simulink model "Uni2Diff"  (R2021b)
settings: Solver=VariableStepAuto  StartTime=0.0  StopTime=10.0  RelTol=1e-3
settings Model: Creator=ericp  LastModifiedBy=ericp

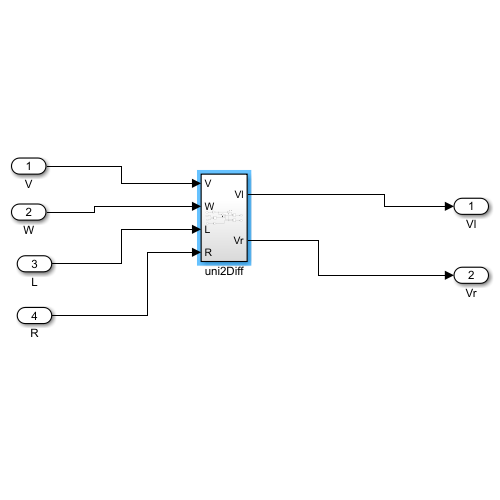
[thumbnail: Simulink's stored preview of the top-level diagram]
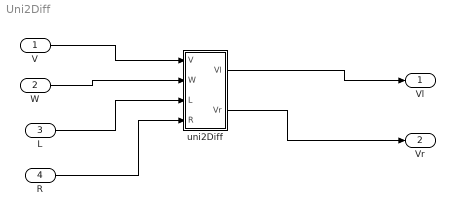
== system Uni2Diff ==
  V : Inport
  W : Inport  Port=2
  L : Inport  Port=3
  R : Inport  Port=4
  uni2Diff : Subsystem
  Vl : Outport
  Vr : Outport  Port=2
  wires:
  V/1 -> uni2Diff/1(V)
  W/1 -> uni2Diff/2(W)
  L/1 -> uni2Diff/3(L)
  R/1 -> uni2Diff/4(R)
  uni2Diff/1(Vl) -> Vl/1
  uni2Diff/2(Vr) -> Vr/1

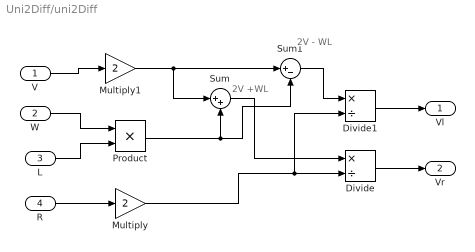
== system Uni2Diff/uni2Diff ==
  note: 2V +WL
  note: 2V - WL
  V : Inport
  W : Inport  Port=2
  L : Inport  Port=3
  R : Inport  Port=4
  Divide : Product  Inputs=*/
  Divide1 : Product  Inputs=*/
  Multiply : Gain  Gain=2
  Multiply1 : Gain  Gain=2
  Product : Product
  Sum : Sum  Inputs=|++
  Sum1 : Sum  Inputs=|+-
  Vl : Outport
  Vr : Outport  Port=2
  wires:
  V/1 -> Multiply1/1
  Divide/1 -> Vr/1
  Sum1/1 -> Divide1/1
  Multiply/1 -> Divide1/2, Divide/2
  Divide1/1 -> Vl/1
  L/1 -> Product/2
  R/1 -> Multiply/1
  Multiply1/1 -> Sum1/1, Sum/1
  Sum/1 -> Divide/1
  Product/1 -> Sum1/2, Sum/2
  W/1 -> Product/1
